simulink library "BeamStressLib"  (R2020a)
settings: Solver=VariableStepAuto  StartTime=0.0  StopTime=10.0  RelTol=1e-3
undefined symbols (not defined in the file): X, Y, Z
libraries: nesl_utility x16, sm_lib x9, sharedtransform x3
(part 1 of 2)
settings Model: Creator=mora  LastModifiedBy=mora

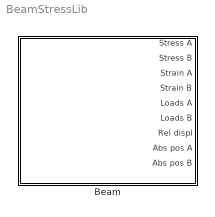
== system BeamStressLib ==
  Beam : Subsystem  mask(This block is a dynamic model of flexible beams with a stress estimation.){E=0, nu=0, rho=0, beta=0, L=0, b=0, h=0, Parameter17=on, Parameter18=on, Parameter13=off, Parameter14=off, FlagPlotStress=off, TimeStartPlot=99.99, BeamID=1, Indx_BandedOrSmooth=Banded, N_elements=1, BeamColor=[0.5 0.5 0.5], Opacity=1}
      mask prompts: E "Young modulus [MPa]"; nu "Poisson ratio [m/m]"; rho "Density [kg/m³]"; beta "Proport damping stiff const (beta) [s]"; L "Length L [m]"; b "Width b [m]"; h "Heigth h [m]"; Parameter17 "Get stress at beam ends [MPa]"; Parameter18 "Get strain at beam ends [m/m]"; Parameter13 "Get forces at beam ends [N] and [N*m]"; Parameter14 "Get beam relative displacements [m] and [rad]"; FlagPlotStress "Plot stress with embedded function (Press "Apply" to update mask)"; TimeStartPlot "Time from start plot stresses [s]"; BeamID "Beam ID numer"; Indx_BandedOrSmooth "Plot color contours appearence"; N_elements "Number of elements"; BeamColor "Beam Color"
      mask help: This block use "General Flexible Beam" of Simscape for rappresent static and dynamic behaviour of flexible elements with generic rectangular cross-section, estimating the stress at its ends.
      mask init:
      | %% Hide and show the parameters of plot stress
      | p=Simulink.Mask.get(gcb);
      | if FlagPlotStress==1
      |     p.getDialogControl('Container22').Visible='on';
      | else
      |     p.getDialogControl('Container22').Visible='off';
      | end
      mask Help:
      | Simscape is a powerful tool embedded in Simulink environment that helps you to model physical systems. Simscape multubody give the possibility to model flexible beams using Euler theory. However, in engineering problems, it is very common to design and optimize structural elements, and for this reason it is important to keep under control the stress in the structure. Simscape library does not provide such important information (and moreover it is not easy to extract information like displacements or forces).
      | The aim of this library is to expand Simscape beam library, providing all the information an engineer requires, in a straightforward way.
      | 
      | This block relies on Simscape "General Flexible Beam" to represent static and dynamic behaviour of flexible beam, with a rectangular cross-section, estimating the stress (and other results) at its ends. The flexible element used is "General Flexible Beam" of Simscape library in order to be compatible also with Simscape releases before 2020a.
      | 
      | A routine helps you to visualize the stress data and better understanding the stress distribution in the cross section. You can turn on and off the visualization routine in the "Output Parameters" tab.
      | IMPORTANT: stresses are computed only on 9 points in the cross section. The plot adopts a linear interpolation between those points just to better visualize, with some approximation, the stress distribution.
      | 
      | The nine points of the cross-section considered are the following:
      | 
      |                                            ↑ y
      |                                             |
      |                                             |
      |                 B                      E |                         A
      |                   *-----------------*-----------------*         --------
      |                   |                         |                       |                 ↑
      |                   |                         |                       |                  |
      |                   |                         |                       |                  |
      |                   |                         |                       |          x      |
      |                F *                       *----------------* H ----→   h
      |                   |                      I                          |                 |
      |                   |                                                 |                  |
      |                   |                                                 |                  |
      |                   |                                                 |                 ↓
      |                   *-----------------*-----------------*         --------
      |                 C                       G                        D
      | 
      |                   |                                                   |
      |                   |                                                   |
      |                   ⇤----------------b-----------------⇥
      | 
      | 
      | This custom block allows you to input geometry, material of the beam, and when you connect the two ports of the beam to the rest of the world, it computes stress, strain displacement and applied loads on the beam ends. Data refer to the International System of Units (m, rad, s) even if the Young modulus E and the stress are measured in MPa (and not Pa), as in the usual practice.
      | 
      | Stresses are evaluated keeping into account both bending stress, normal stress, shear stress and torsional stress in 9 different points of the cross-section of the beam (at the four edges, four in the middle of each side and one in the center of the beam). Stresses are combined according to Von-Mises equivalent stress. The stress analysis, as well as the Simscape beam model (General Flexible Beam), assume the beam is “long”, in comparison to the cross-section, adopting Euler-theory where the bending effect is greater than shear effect (i.e. shear compliance is neglected). In other words, the length of the beam should be about x10 times the cross-section side. Only for short beams shear deflection is not negligible and therefore it is better to use Timoshenko-Ehrenfest beam theory (at the moment not implemented in Simscape).
      | 
      | The results of this library were checked with a professional FEM software, showing a good agreement.
      mask TypeOptions Indx_BandedOrSmooth: Banded | Smooth
      mask DialogControl Control4 Tooltip: Main element of the beam
      mask DialogControl Container9 Prompt: Input parameters
      mask DialogControl MaterialGroupVar Prompt: Material
      mask DialogControl GeometryGroupVar Prompt: Geometry
      mask DialogControl Container18 Prompt: Output parameters
      mask DialogControl Container22 Prompt: Plot settings
      mask DialogControl Container19 Prompt: Plot help
      mask DialogControl Control2 Prompt: Since plotting the stress of the two ends is time consuming task, it is better to plot stress only at the end of the simulation, when the structure is fully loaded. Therefore it is advisable to use a "Time from start to plot stresses" close to the simulation time. For example: simulation time = 10 s, time from start plot stresses = 9.99 s. In this way the plot routine is invoke only in the few last time step without slowing down the computational time of the simulation. In order to distinguish the stress of each beam, a unique ID number is provided.
      mask DialogControl Container8 Prompt: Advanced options
      mask DialogControl Container12 Prompt: Discretization
      mask DialogControl Container13 Prompt: Graphic
      mask Display: image('$imagefile'); % Use "Edit Image" on toolstrip to change.

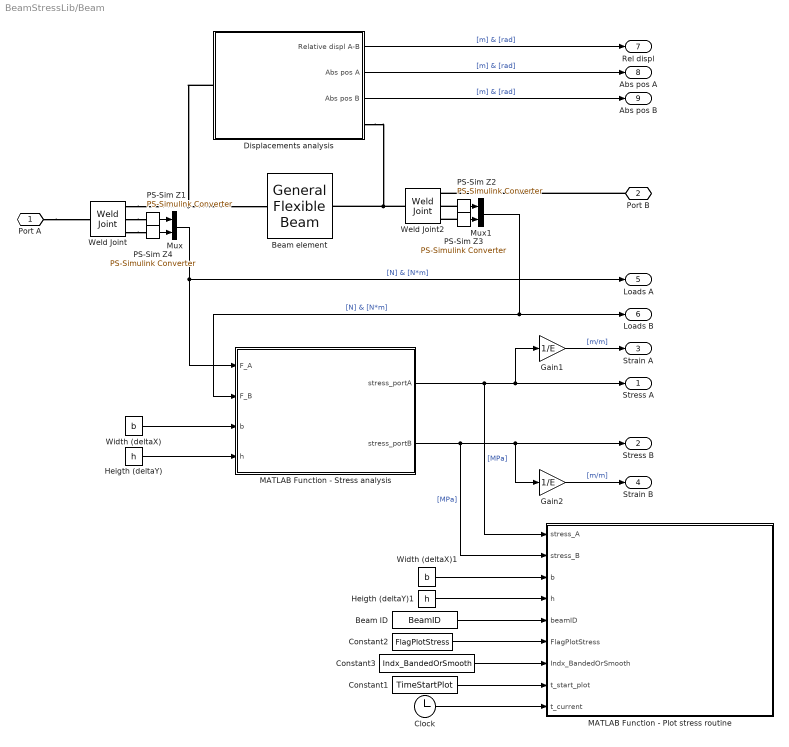
== system BeamStressLib/Beam ==
  Beam ID : Constant  Value=BeamID
  Beam element : sm_lib/Body Elements/Flexible Bodies/Beams/General Flexible Beam  GraphicAmbientColor=[0.15 0.15 0.15 1.0]  GraphicDiffuseColor=BeamColor  ExtrusionCrossSection=[b h; -b h; -b -h; b -h]/2  ExtrusionCrossSectionUnits=m  DampingType=Proportional  Density=rho  DensityUnits=kg/m^3  GraphicEmissiveColor=[0.0 0.0 0.0 1.0]  GraphicType=FromGeometry  ExtrusionLength=L  ExtrusionLengthUnits=m  ModuliType=YoungsPoissons  NumElements=N_elements  GraphicOpacity=Opacity  PoissonsRatio=.3  ShearModulus=26  ShearModulusUnits=GPa  GraphicShininess=75  GraphicSpecularColor=[0.5 0.5 0.5 1.0]  StiffnessType=FromGeometry  GraphicVisPropType=SimpleVisualProperties  YoungsModulus=E  YoungsModulusUnits=MPa  ProportionalDampingAlpha=0  ProportionalDampingAlphaUnits=1/s  ProportionalDampingBeta=dampingConstant  ProportionalDampingBetaUnits=s  UniformModalDampingRatio=0.01
      settings: SourceProductBaseCode=MS
  Clock : Clock
  Constant1 : Constant  Value=TimeStartPlot
  Constant2 : Constant  Value=FlagPlotStress
  Constant3 : Constant  Value=Indx_BandedOrSmooth
  Displacements analysis : Subsystem
      mask Display: image('$imagefile'); % Use "Edit Image" on toolstrip to change.
  Gain1 : Gain  Gain=1/E
  Gain2 : Gain  Gain=1/E
  Heigth (deltaY) : Constant  Value=h
  Heigth (deltaY)1 : Constant  Value=h
  MATLAB Function - Plot stress routine : MATLAB Function  TreatAsAtomicUnit=on
  MATLAB Function - Stress analysis : MATLAB Function  TreatAsAtomicUnit=on
  Mux : Mux  Inputs=2
  Mux1 : Mux  Inputs=2
  PS-Sim Z{1..4} (4 alike) : nesl_utility/PS-Simulink Converter  PhysicalDomain=network_engine_domain  SubClassName=ps_output  LeftPortType=input  RightPortType=output  PseudoPeriodic=off  Frequencies=[]  Unit=1  AffineConversion=off
  Weld Joint : sm_lib/Joints/Weld Joint  JointMode=Normal  SenseConstraintForce=on  SenseConstraintForceX=off  SenseConstraintForceY=off  SenseConstraintForceZ=off  SenseConstraintTorque=on  SenseConstraintTorqueX=off  SenseConstraintTorqueY=off  SenseConstraintTorqueZ=off  SenseTotalForce=off  SenseTotalForceX=off  SenseTotalForceY=off  SenseTotalForceZ=off  SenseTotalTorque=off  SenseTotalTorqueX=off  SenseTotalTorqueY=off  SenseTotalTorqueZ=off  CompositeWrenchDir=BaseOnFollower  CompositeWrenchFrame=FollowerFrame
  Weld Joint2 : sm_lib/Joints/Weld Joint  JointMode=Normal  SenseConstraintForce=on  SenseConstraintForceX=off  SenseConstraintForceY=off  SenseConstraintForceZ=off  SenseConstraintTorque=on  SenseConstraintTorqueX=off  SenseConstraintTorqueY=off  SenseConstraintTorqueZ=off  SenseTotalForce=off  SenseTotalForceX=off  SenseTotalForceY=off  SenseTotalForceZ=off  SenseTotalTorque=off  SenseTotalTorqueX=off  SenseTotalTorqueY=off  SenseTotalTorqueZ=off  CompositeWrenchDir=FollowerOnBase  CompositeWrenchFrame=BaseFrame
  Width (deltaX) : Constant  Value=b
  Width (deltaX)1 : Constant  Value=b
  Port A : PMIOPort  Side=Left
  Port B : PMIOPort  Port=2  Side=Right
  Stress A : Outport  VectorParamsAs1DForOutWhenUnconnected=off
  Stress B : Outport  Port=2  VectorParamsAs1DForOutWhenUnconnected=off
  Strain A : Outport  Port=3  VectorParamsAs1DForOutWhenUnconnected=off
  Strain B : Outport  Port=4  VectorParamsAs1DForOutWhenUnconnected=off
  Loads A : Outport  Port=5  VectorParamsAs1DForOutWhenUnconnected=off
  Loads B : Outport  Port=6  VectorParamsAs1DForOutWhenUnconnected=off
  Rel displ : Outport  Port=7  VectorParamsAs1DForOutWhenUnconnected=off
  Abs pos A : Outport  Port=8  VectorParamsAs1DForOutWhenUnconnected=off
  Abs pos B : Outport  Port=9  VectorParamsAs1DForOutWhenUnconnected=off
  wires:
  Heigth (deltaY)/1 -> MATLAB Function - Stress analysis/4(h)
  MATLAB Function - Stress analysis/2(stress_portB) -> MATLAB Function - Plot stress routine/2(stress_B), Gain2/1, Stress B/1  "[MPa]"
  Width (deltaX)/1 -> MATLAB Function - Stress analysis/3(b)
  Displacements analysis/1(Relative displ A-B) -> Rel displ/1  "[m] & [rad]"
  PS-Sim Z1/1 -> Mux/1
  PS-Sim Z4/1 -> Mux/2
  Mux/1 -> MATLAB Function - Stress analysis/1(F_A), Loads A/1  "[N] & [N*m]"
  PS-Sim Z2/1 -> Mux1/1
  PS-Sim Z3/1 -> Mux1/2
  Mux1/1 -> MATLAB Function - Stress analysis/2(F_B), Loads B/1  "[N] & [N*m]"
  Gain1/1 -> Strain A/1  "[m/m]"
  Gain2/1 -> Strain B/1  "[m/m]"
  Displacements analysis/2(Abs pos A) -> Abs pos A/1  "[m] & [rad]"
  Displacements analysis/3(Abs pos B) -> Abs pos B/1  "[m] & [rad]"
  Width (deltaX)1/1 -> MATLAB Function - Plot stress routine/3(b)
  Heigth (deltaY)1/1 -> MATLAB Function - Plot stress routine/4(h)
  Beam ID/1 -> MATLAB Function - Plot stress routine/5(beamID)
  Constant2/1 -> MATLAB Function - Plot stress routine/6(FlagPlotStress)
  MATLAB Function - Stress analysis/1(stress_portA) -> MATLAB Function - Plot stress routine/1(stress_A), Gain1/1, Stress A/1  "[MPa]"
  Constant1/1 -> MATLAB Function - Plot stress routine/8(t_start_plot)
  Clock/1 -> MATLAB Function - Plot stress routine/9(t_current)
  Constant3/1 -> MATLAB Function - Plot stress routine/7(Indx_BandedOrSmooth)
  connections:
  Port A/RConn1 -- Weld Joint/LConn1
  Port B/RConn1 -- Weld Joint2/RConn1
  PS-Sim Z3/LConn1 -- Weld Joint2/RConn3
  PS-Sim Z2/LConn1 -- Weld Joint2/RConn2
  Weld Joint/RConn1 -- Displacements analysis/LConn1 -- Beam element/LConn1
  Weld Joint2/LConn1 -- Displacements analysis/RConn1 -- Beam element/RConn1
  Weld Joint/RConn2 -- PS-Sim Z1/LConn1
  Weld Joint/RConn3 -- PS-Sim Z4/LConn1

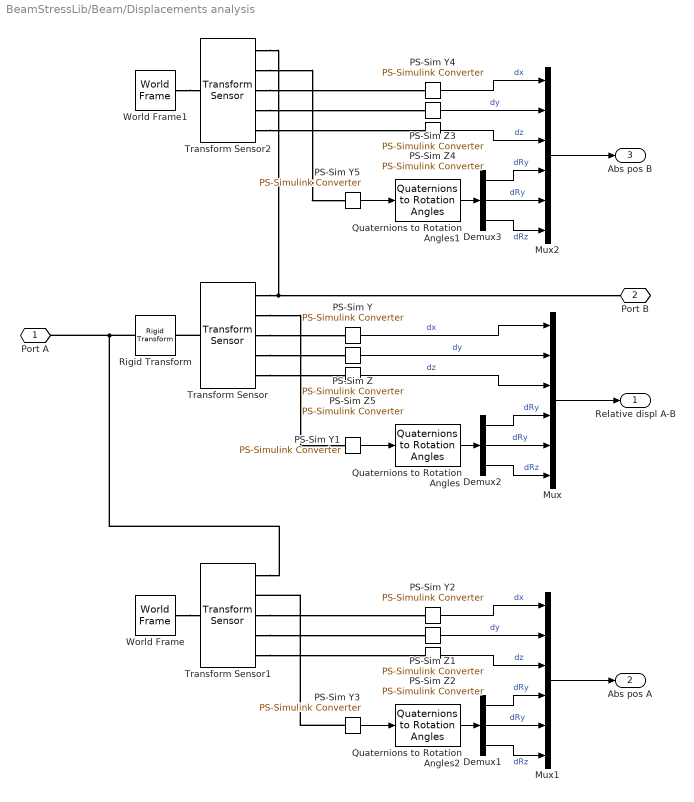
== system BeamStressLib/Beam/Displacements analysis ==
  Demux1 : Demux  Outputs=3
  Demux2 : Demux  Outputs=3
  Demux3 : Demux  Outputs=3
  Mux : Mux  Inputs=6
  Mux1 : Mux  Inputs=6
  Mux2 : Mux  Inputs=6
  PS-Sim Y{,1..5} (6 alike) : nesl_utility/PS-Simulink Converter  PhysicalDomain=network_engine_domain  SubClassName=ps_output  LeftPortType=input  RightPortType=output  PseudoPeriodic=off  Frequencies=[]  Unit=1  AffineConversion=off
  PS-Sim Z{,1..5} (6 alike) : nesl_utility/PS-Simulink Converter  PhysicalDomain=network_engine_domain  SubClassName=ps_output  LeftPortType=input  RightPortType=output  PseudoPeriodic=off  Frequencies=[]  Unit=1  AffineConversion=off
  Quaternions to Rotation Angles : sharedtransform/Quaternions to Rotation Angles  rotationOrder=XYZ  aMode=aMode
      settings: SourceProductBaseCode=AE,PW,MT,VE,VP
  Quaternions to Rotation Angles1 : sharedtransform/Quaternions to Rotation Angles  rotationOrder=XYZ  aMode=aMode
      settings: SourceProductBaseCode=AE,PW,MT,VE,VP
  Quaternions to Rotation Angles2 : sharedtransform/Quaternions to Rotation Angles  rotationOrder=XYZ  aMode=aMode
      settings: SourceProductBaseCode=AE,PW,MT,VE,VP
  Rigid Transform : sm_lib/Frames and Transforms/Rigid Transform  TranslationMethod=StandardAxis  TranslationStandardOffset=L  TranslationLengthUnit=m  TranslationStandardAxis=+Z  TranslationCartesianOffset=[0 0 0]  TranslationROffset=0  TranslationROffsetUnits=m  TranslationZOffset=0  TranslationZOffsetUnits=m  TranslationThetaOffset=0  TranslationThetaOffsetUnits=deg  RotationMethod=None  RotationAngleUnits=deg  RotationStandardAxis=+Z  RotationAngle=0.0  RotationArbitraryAxis=[0 0 1]  FollAlignAxisA=+X  BaseAlignAxisA=+Y  FollAlignAxisB=+Y  BaseAlignAxisB=+Z  RotationSequenceAxes=FollowerAxes  RotationSequence=XYX  RotationSequenceAngles=[0 0 0]  RotationSequenceAnglesUnits=deg  RotationMatrix=[1 0 0; 0 1 0; 0 0 1]
  Transform Sensor : sm_lib/Frames and Transforms/Transform Sensor  MeasurementFrame=World  SenseAngle=off  SenseAxis=off  SenseAngle1=off  SenseAngle2=off  SenseAngle3=off  SenseQ=on  SenseR=off  SenseOmegaX=off  SenseOmegaY=off  SenseOmegaZ=off  SenseOmega1=off  SenseOmega2=off  SenseOmega3=off  SenseQDot=off  SenseRDot=off  SenseAlphaX=off  SenseAlphaY=off  SenseAlphaZ=off  SenseAlpha1=off  SenseAlpha2=off  SenseAlpha3=off  SenseQDDot=off  SenseRDDot=off  SenseX=on  SenseY=on  SenseZ=on  SenseRad=off  SenseAzim=off  SenseDist=off  SenseInc=off  SenseXDot=off  SenseYDot=off  SenseZDot=off  SenseRadDot=off  SenseAzimDot=off  SenseDistDot=off  SenseIncDot=off  SenseXDDot=off  SenseYDDot=off  SenseZDDot=off  SenseRadDDot=off  SenseAzimDDot=off  SenseDistDDot=off  SenseIncDDot=off
  Transform Sensor1 : sm_lib/Frames and Transforms/Transform Sensor  MeasurementFrame=World  SenseAngle=off  SenseAxis=off  SenseAngle1=off  SenseAngle2=off  SenseAngle3=off  SenseQ=on  SenseR=off  SenseOmegaX=off  SenseOmegaY=off  SenseOmegaZ=off  SenseOmega1=off  SenseOmega2=off  SenseOmega3=off  SenseQDot=off  SenseRDot=off  SenseAlphaX=off  SenseAlphaY=off  SenseAlphaZ=off  SenseAlpha1=off  SenseAlpha2=off  SenseAlpha3=off  SenseQDDot=off  SenseRDDot=off  SenseX=on  SenseY=on  SenseZ=on  SenseRad=off  SenseAzim=off  SenseDist=off  SenseInc=off  SenseXDot=off  SenseYDot=off  SenseZDot=off  SenseRadDot=off  SenseAzimDot=off  SenseDistDot=off  SenseIncDot=off  SenseXDDot=off  SenseYDDot=off  SenseZDDot=off  SenseRadDDot=off  SenseAzimDDot=off  SenseDistDDot=off  SenseIncDDot=off
  Transform Sensor2 : sm_lib/Frames and Transforms/Transform Sensor  MeasurementFrame=World  SenseAngle=off  SenseAxis=off  SenseAngle1=off  SenseAngle2=off  SenseAngle3=off  SenseQ=on  SenseR=off  SenseOmegaX=off  SenseOmegaY=off  SenseOmegaZ=off  SenseOmega1=off  SenseOmega2=off  SenseOmega3=off  SenseQDot=off  SenseRDot=off  SenseAlphaX=off  SenseAlphaY=off  SenseAlphaZ=off  SenseAlpha1=off  SenseAlpha2=off  SenseAlpha3=off  SenseQDDot=off  SenseRDDot=off  SenseX=on  SenseY=on  SenseZ=on  SenseRad=off  SenseAzim=off  SenseDist=off  SenseInc=off  SenseXDot=off  SenseYDot=off  SenseZDot=off  SenseRadDot=off  SenseAzimDot=off  SenseDistDot=off  SenseIncDot=off  SenseXDDot=off  SenseYDDot=off  SenseZDDot=off  SenseRadDDot=off  SenseAzimDDot=off  SenseDistDDot=off  SenseIncDDot=off
  World Frame : sm_lib/Frames and Transforms/World Frame
  World Frame1 : sm_lib/Frames and Transforms/World Frame
  Port A : PMIOPort  Side=Left
  Port B : PMIOPort  Port=2  Side=Right
  Relative displ A-B : Outport  VectorParamsAs1DForOutWhenUnconnected=off
  Abs pos A : Outport  Port=2  VectorParamsAs1DForOutWhenUnconnected=off
  Abs pos B : Outport  Port=3  VectorParamsAs1DForOutWhenUnconnected=off
  wires:
  PS-Sim Z/1 -> Mux/2  "dy"
  PS-Sim Z5/1 -> Mux/3  "dz"
  PS-Sim Y/1 -> Mux/1  "dx"
  Mux/1 -> Relative displ A-B/1
  PS-Sim Z2/1 -> Mux1/3  "dz"
  PS-Sim Z1/1 -> Mux1/2  "dy"
  PS-Sim Y2/1 -> Mux1/1  "dx"
  Mux1/1 -> Abs pos A/1
  Mux2/1 -> Abs pos B/1
  PS-Sim Y4/1 -> Mux2/1  "dx"
  PS-Sim Z3/1 -> Mux2/2  "dy"
  PS-Sim Z4/1 -> Mux2/3  "dz"
  Demux2/1 -> Mux/4  "dRy"
  Demux2/2 -> Mux/5  "dRy"
  Demux2/3 -> Mux/6  "dRz"
  Quaternions to Rotation Angles/1 -> Demux2/1
  PS-Sim Y1/1 -> Quaternions to Rotation Angles/1
  Demux3/3 -> Mux2/6  "dRz"
  Demux3/2 -> Mux2/5  "dRy"
  Demux3/1 -> Mux2/4  "dRy"
  PS-Sim Y5/1 -> Quaternions to Rotation Angles1/1
  Quaternions to Rotation Angles1/1 -> Demux3/1
  Demux1/3 -> Mux1/6  "dRz"
  Demux1/2 -> Mux1/5  "dRy"
  Demux1/1 -> Mux1/4  "dRy"
  PS-Sim Y3/1 -> Quaternions to Rotation Angles2/1
  Quaternions to Rotation Angles2/1 -> Demux1/1
  connections:
  Transform Sensor/LConn1 -- Rigid Transform/RConn1
  Transform Sensor/RConn1 -- Port B/RConn1 -- Transform Sensor2/RConn1
  Rigid Transform/LConn1 -- Transform Sensor1/RConn1 -- Port A/RConn1
  World Frame/RConn1 -- Transform Sensor1/LConn1
  Transform Sensor1/RConn5 -- PS-Sim Z2/LConn1
  Transform Sensor1/RConn4 -- PS-Sim Z1/LConn1
  Transform Sensor1/RConn3 -- PS-Sim Y2/LConn1
  Transform Sensor2/RConn3 -- PS-Sim Y4/LConn1
  Transform Sensor2/RConn4 -- PS-Sim Z3/LConn1
  Transform Sensor2/RConn5 -- PS-Sim Z4/LConn1
  World Frame1/RConn1 -- Transform Sensor2/LConn1
  Transform Sensor/RConn2 -- PS-Sim Y1/LConn1
  Transform Sensor/RConn3 -- PS-Sim Y/LConn1
  Transform Sensor/RConn4 -- PS-Sim Z/LConn1
  Transform Sensor/RConn5 -- PS-Sim Z5/LConn1
  Transform Sensor2/RConn2 -- PS-Sim Y5/LConn1
  PS-Sim Y3/LConn1 -- Transform Sensor1/RConn2

== matlab function BeamStressLib/Beam/MATLAB Function - Plot stress routine ==
  data: stress_A input; stress_B input; b input; h input; beamID input; FlagPlotStress input; Indx_BandedOrSmooth input; t_start_plot input; t_current input
function fcn(stress_A, stress_B, b, h, beamID, FlagPlotStress, Indx_BandedOrSmooth, t_start_plot, t_current)
%%%%%%%%%%%%%%%%%%%%%%%%%%%%%%%%%%%%%%%%%%%%%%%%%%%%%%%%%%%%%%%%%%%%%%%%%%%
% INPUTS:
%            stress_A = Stress signal with 9 components for port A of the beam.
%
%            stress_B = Stress signal with 9 components for port B of the beam.
%
%                   b = Width of the beam (in x direction!).
%                       This is NOT strictly smaller than h.
%
%                   h = Heigth of the beam (in y direction!).
%                       This is NOT strictly bigger than b.
%
%              beamID = Unique constant number that distinguish the beam under
%                       analysis to the other beams in the model.
%
%      FlagPlotStress = Bool value from the checkbox of the mask of this 
%                       library (Output settings).
%
% Indx_BandedOrSmooth = Value from the popup of the mask (Output settings) that decide the
%                       appearence of the stress plot.
%                       Indx_BandedOrSmooth = 1   ->  banded plot (low color levels)
%                       Indx_BandedOrSmooth = 2   ->  smooth plot (high color levels)
%
%        t_start_plot = Value set from the mask (Output settings). When
%                       t_current>t_start_plot, the stress graph is plotted.
%
%           t_current = Current time of the simulation.
% 
%%%%%%%%%%%%%%%%%%%%%%%%%%%%%%%%%%%%%%%%%%%%%%%%%%%%%%%%%%%%%%%%%%%%%%%%%%%
% OUTPUTS:
%       One figure for each beam ID with two subplot: the upper subplot
%       rappresent the stress at port A, the lower subplot rappresent the
%       stress at port B.
%
%
%%%%%%%%%%%%%%%%%%%%%%%%%%%%%%%%%%%%%%%%%%%%%%%%%%%%%%%%%%%%%%%%%%%%%%%%%%%
% HYPOTESIS and NOTES:
%
%  0) We compute stresses only for generic beams with rectangular (or squared)
%     cross section.
%  1) The stress of this routine are check with NX Nastran FEM software by
%     the author using a 1D beam model with generic loading (lumped force
%     and moments, in ordet to validate the goodness of the results.
%     The present routine give results in good agreement with sthe FEM model.
%
%
%  In particular
%  - the 1st element (named A) is point with coordinate [+b/2 +h/2]
%  - the 2nd element (named B) is point with coordinate [-b/2 +h/2]
%  - the 3rd element (named C) is point with coordinate [-b/2 -h/2]
%  - the 4th element (named D) is point with coordinate [+b/2 -h/2]
%  - the 5th element (named E) is point with coordinate [  0  +h/2]
%  - the 6th element (named F) is point with coordinate [-b/2   0 ]
%  - the 7th element (named G) is point with coordinate [  0  -h/2]
%  - the 8th element (named H) is point with coordinate [+b/2   0 ]
%  - the 9th element (named I) is point with coordinate [  0    0 ]
%
%
% Cross section view of the beam.
%                                   ↑ y
%                                   |
%                                   |
%                  B               E|                A
%                   *---------------*---------------*            ----
%                   |               |               |               ↑
%                   |               |               |               |
%                   |               |               |               |
%                   |               |               |        x      |
%                 F *               *---------------* H ----→      h
%                   |              I                |               |
%                   |                               |               |
%                   |                               |               |
%                   |                               |               ↓
%                   *---------------*---------------*            ----
%                  C               G                 D
%
%                   |                               |
%                   |                               |
%                   ⇤--------------b---------------⇥
%
%  
%%%%%%%%%%%%%%%%%%%%%%%%%%%%%%%%%%%%%%%%%%%%%%%%%%%%%%%%%%%%%%%%%%%%%%%%%%%
% Author: Alberto Mora, (STIIMA - CNR)   http://www.stiima.cnr.it/en/
% Date:   26/05/2020
%%%%%%%%%%%%%%%%%%%%%%%%%%%%%%%%%%%%%%%%%%%%%%%%%%%%%%%%%%%%%%%%%%%%%%%%%%%
% REVISION:
%       v0.0   First release
%%%%%%%%%%%%%%%%%%%%%%%%%%%%%%%%%%%%%%%%%%%%%%%%%%%%%%%%%%%%%%%%%%%%%%%%%%% 
%% Set special coder settings allows plot of stress
coder.extrinsic('round');
coder.extrinsic('range');
coder.extrinsic('colorbar');                                                % Enable colorbar in MATLAB function (disable by default),
                                                                            % see https://it.mathworks.com/matlabcentral/answers/542012-colorbar-not-supported-in-simulink-matlab-function-surf-plot

if t_current>t_start_plot && FlagPlotStress                                 % Check if at current iteration we have to plot stress
    %% Prepare data
    X = [ -b  0  b
          -b  0  b
          -b  0  b]/2;                                                      % Create point matrix of y coordinate

    Y = [ -h -h -h
           0  0  0
           h  h  h]/2;                                                      % Create point matrix of y coordinate

    Z_A=[ stress_A(3) stress_A(7) stress_A(4)
          stress_A(6) stress_A(9) stress_A(8)
          stress_A(2) stress_A(5) stress_A(1)];                             % Create stress matrix for port A
    
    IndxMaxStress_A = find(max(Z_A(:))==Z_A);                               % Find the point with highest stress.
    IndxMaxStress_A = IndxMaxStress_A(1);                                   % If there are multiple poit with the same max stress, choose the first. For example, in pure bending, the side has same max stress on all 3 points.
    
    Z_B=[ stress_B(3) stress_B(7) stress_B(4)
          stress_B(6) stress_B(9) stress_B(8)
          stress_B(2) stress_B(5) stress_B(1)];                             % Create stress matrix for port B
      
    IndxMaxStress_B = find(max(Z_B(:))==Z_B);                               % Find the point with highest stress.
    IndxMaxStress_B = IndxMaxStress_B(1);                                   % If there are multiple poit with the same max stress, choose the first. For example, in pure bending, the side has same max stress on all 3 points.
    
    
    %% Parameters for the plot
    ColorLevel=0;                                                           % Initialize ColorLevel
    % Number of color division of the surf plot. Choose low for banded, choose high value for smooth.
    if Indx_BandedOrSmooth==1
        ColorLevel=12;                                                      % Banded
    elseif Indx_BandedOrSmooth==2
        ColorLevel=150;                                                     % Smooth
    end
    
    InterpolationPoints=20;                                                 % Points for the 2D-interpolation of the surf plot refinement. Must be odd.
    InterpolationPoints=2*floor(InterpolationPoints/2)+1;                   % Just for safety, to be sure to get odd number...
    
    Colorbar_N_ScaleDivision = 7;                                           % Number of division of the colorbar scale
    Colorbar_NumberDigits = 2;                                              % Digits after comma of the colorbar numbers
    
    LettersArray = ['C','G','D';
                    'F','I','H';
                    'B','E','A'];
    
    % Set proper color to each letter - PORT A
    LetterColor_A={'','','','','','','','',''};
    for n=1:length(Z_A(:))                                                  % Choose color of letters, according to the surf color. If the surf is yellow or green, we choose black letter, otherwise we choose white letters
        if Z_A(n)-min(Z_A(:))>0.3*(max(Z_A(:))-min(Z_A(:)))   &&   Z_A(n)-min(Z_A(:))<0.75*(max(Z_A(:))-min(Z_A(:)))
            LetterColor_A{n}='black';
        else
            LetterColor_A{n}='white';
        end
    end
    
    % Set proper color to each letter - PORT B
    LetterColor_B={'','','','','','','','',''};
    for n=1:length(Z_B(:))                                                  % Choose color of letters, according to the surf color. If the surf is yellow or green, we choose black letter, otherwise we choose white letters
        if Z_B(n)-min(Z_B(:))>0.3*(max(Z_B(:))-min(Z_B(:)))   &&   Z_B(n)-min(Z_B(:))<0.75*(max(Z_B(:))-min(Z_B(:)))
            LetterColor_B{n}='black';
        else
            LetterColor_B{n}='white';
        end
    end
    
    
    %% Main computations
    [X_interp,Y_interp] = meshgrid(linspace(-b,b,InterpolationPoints)/2,linspace(-h,h,InterpolationPoints)/2);
    Z_interp_A = interp2(X,Y,Z_A,X_interp,Y_interp,'linear');
    Z_interp_B = interp2(X,Y,Z_B,X_interp,Y_interp,'linear');
    
    
    %% Plot
    
    figure(beamID)                                                          % Overwrite the new plot on the correct figure of the correct beam ID
    subplot(2,1,1);
    surf(X_interp,Y_interp,Z_interp_A,'FaceColor','interp','EdgeColor','none');hold on;
    mesh(X,Y,Z_A,'FaceColor','none','EdgeColor','k'); hold off;
%     text(X(IndxMaxStress_A),Y(IndxMaxStress_A),max(Z_A(:)),'O','HorizontalAlignment','center','FontSize',14);
%     text(X(IndxMaxStress_A),Y(IndxMaxStress_A),max(Z_A(:)),sprintf('  Max stress = %.1f MPa',max(Z_A(:))),'HorizontalAlignment','left','VerticalAlignment','bottom','FontSize',10);
    text(-b/2, h*0.6, sprintf('Current plot time = %.3f s',t_current) );
    asp_ratio = daspect; daspect([1 1 asp_ratio(3)]); colormap(jet(ColorLevel)); box on; view(2);
    xlabel('x_{beam} [m]'); ylabel('y_{beam} [m]'); zlabel('\sigma_{Von-Mises} [MPa]');
    title({sprintf('Beam ID = %d ', int32(beamID));
            ['\fontsize{9}',sprintf('Port A - Max von Mises stress = %.2f MPa',max(Z_A(:))),' at point ',LettersArray(IndxMaxStress_A)']});
    ValForColorbar = round(linspace(min(Z_A(:)),max(Z_A(:)),Colorbar_N_ScaleDivision),Colorbar_NumberDigits);
    colorbar('Ticks',[ValForColorbar(1)*1.01 ValForColorbar(2:Colorbar_N_ScaleDivision-1)   ValForColorbar(Colorbar_N_ScaleDivision)*0.99],...% Move sligly high the lower stress to avoid numerical problems (value not shown)
            'TickLabels',ValForColorbar);                                   % Print on colorbar the correct values
    n=1; text(X(n)*0.98,Y(n),max(Z_A(:))*1.2, LettersArray(n),'Color',LetterColor_A{n},'HorizontalAlignment','left', 'VerticalAlignment','bottom');%C
    n=2; text(X(n)*0.98,Y(n),max(Z_A(:))*1.2, LettersArray(n),'Color',LetterColor_A{n},'HorizontalAlignment','left', 'VerticalAlignment','bottom');%F
    n=3; text(X(n)*0.98,Y(n),max(Z_A(:))*1.2, LettersArray(n),'Color',LetterColor_A{n},'HorizontalAlignment','left', 'VerticalAlignment','top'   );%B
    n=4; text(X(n)     ,Y(n),max(Z_A(:))*1.2, LettersArray(n),'Color',LetterColor_A{n},'HorizontalAlignment','left', 'VerticalAlignment','bottom');%G
    n=5; text(X(n)     ,Y(n),max(Z_A(:))*1.2, LettersArray(n),'Color',LetterColor_A{n},'HorizontalAlignment','left', 'VerticalAlignment','bottom');%I
    n=6; text(X(n)     ,Y(n),max(Z_A(:))*1.2, LettersArray(n),'Color',LetterColor_A{n},'HorizontalAlignment','left', 'VerticalAlignment','top'   );%E
    n=7; text(X(n)*0.98,Y(n),max(Z_A(:))*1.2, LettersArray(n),'Color',LetterColor_A{n},'HorizontalAlignment','right','VerticalAlignment','bottom');%D
    n=8; text(X(n)*0.98,Y(n),max(Z_A(:))*1.2, LettersArray(n),'Color',LetterColor_A{n},'HorizontalAlignment','right','VerticalAlignment','bottom');%H
    n=9; text(X(n)*0.98,Y(n),max(Z_A(:))*1.2, LettersArray(n),'Color',LetterColor_A{n},'HorizontalAlignment','right','VerticalAlignment','top'   );%A

    subplot(2,1,2);
    surf(X_interp,Y_interp,Z_interp_B,'FaceColor','interp','EdgeColor','none');hold on;
    mesh(X,Y,Z_B,'FaceColor','none','EdgeColor','k'); hold off;
%     text(X(IndxMaxStress_B),Y(IndxMaxStress_B),max(Z_B(:)),'O','HorizontalAlignment','center','FontSize',14);
%     text(X(IndxMaxStress_B),Y(IndxMaxStress_B),max(Z_B(:)),sprintf('  Max stress = %.1f MPa',max(Z_B(:))),'HorizontalAlignment','left','VerticalAlignment','bottom','FontSize',10);
    asp_ratio = daspect; daspect([1 1 asp_ratio(3)]); colormap(jet(ColorLevel));
    xlabel('x_{beam} [m]'); ylabel('y_{beam} [m]'); zlabel('\sigma_{Von-Mises} [MPa]'); box on; view(2);
    title(['\fontsize{9}',sprintf('Port B - Max von Mises stress = %.2f MPa',max(Z_B(:))),' at point ',LettersArray(IndxMaxStress_B)]);
    ValForColorbar = round(linspace(min(Z_B(:)),max(Z_B(:)),Colorbar_N_ScaleDivision),Colorbar_NumberDigits);
    colorbar('Ticks',[ValForColorbar(1)*1.01 ValForColorbar(2:Colorbar_N_ScaleDivision-1)   ValForColorbar(Colorbar_N_ScaleDivision)*0.99],...% Move sligly high the lower stress to avoid numerical problems (value not shown)
            'TickLabels',ValForColorbar);                                   % Print on colorbar the correct values
    n=1; text(X(n)*0.98,Y(n),max(Z_B(:))*1.2, LettersArray(n),'Color',LetterColor_B{n},'HorizontalAlignment','left', 'VerticalAlignment','bottom');%C
    n=2; text(X(n)*0.98,Y(n),max(Z_B(:))*1.2, LettersArray(n),'Color',LetterColor_B{n},'HorizontalAlignment','left', 'VerticalAlignment','bottom');%F
    n=3; text(X(n)*0.98,Y(n),max(Z_B(:))*1.2, LettersArray(n),'Color',LetterColor_B{n},'HorizontalAlignment','left', 'VerticalAlignment','top'   );%B
    n=4; text(X(n)     ,Y(n),max(Z_B(:))*1.2, LettersArray(n),'Color',LetterColor_B{n},'HorizontalAlignment','left', 'VerticalAlignment','bottom');%G
    n=5; text(X(n)     ,Y(n),max(Z_B(:))*1.2, LettersArray(n),'Color',LetterColor_B{n},'HorizontalAlignment','left', 'VerticalAlignment','bottom');%I
    n=6; text(X(n)     ,Y(n),max(Z_B(:))*1.2, LettersArray(n),'Color',LetterColor_B{n},'HorizontalAlignment','left', 'VerticalAlignment','top'   );%E
    n=7; text(X(n)*0.98,Y(n),max(Z_B(:))*1.2, LettersArray(n),'Color',LetterColor_B{n},'HorizontalAlignment','right','VerticalAlignment','bottom');%D
    n=8; text(X(n)*0.98,Y(n),max(Z_B(:))*1.2, LettersArray(n),'Color',LetterColor_B{n},'HorizontalAlignment','right','VerticalAlignment','bottom');%H
    n=9; text(X(n)*0.98,Y(n),max(Z_B(:))*1.2, LettersArray(n),'Color',LetterColor_B{n},'HorizontalAlignment','right','VerticalAlignment','top'   );%A

end
